simulink model "actuatormodel"  (R2019a)
settings: Solver=VariableStepAuto  StartTime=0.0  StopTime=10.0  RelTol=1e-3
settings Model: Creator=sensei  LastModifiedBy=sensei

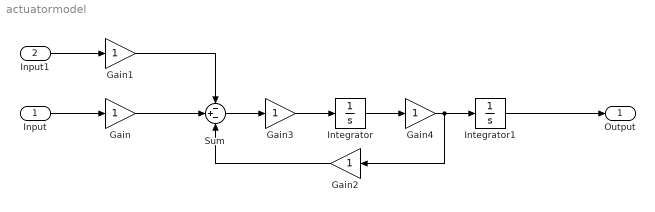
== system actuatormodel ==
  Input : Inport
  Input1 : Inport  Port=2
  Gain{,1..4} (5 alike) : Gain
  Integrator : Integrator
  Integrator1 : Integrator
  Sum : Sum  Inputs=-+-
  Output : Outport
  wires:
  Gain/1 -> Sum/2
  Gain1/1 -> Sum/1
  Input/1 -> Gain/1
  Input1/1 -> Gain1/1
  Sum/1 -> Gain3/1
  Gain2/1 -> Sum/3
  Gain3/1 -> Integrator/1
  Integrator/1 -> Gain4/1
  Gain4/1 -> Gain2/1, Integrator1/1
  Integrator1/1 -> Output/1
